simulink model "traffic_light"  (R2020a)
settings: Solver=VariableStepAuto  StartTime=0.0  StopTime=150  RelTol=1e-3
undefined symbols (not defined in the file): DiscIntNeverNeededParam
libraries: simulink x1
settings Model: Creator=Shubham  LastModifiedBy=Shubham

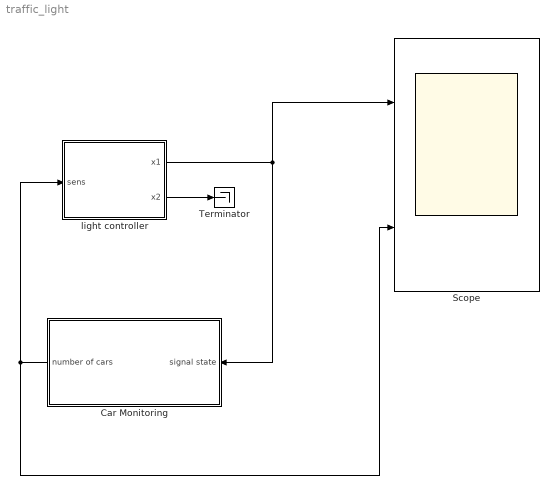
== system traffic_light ==
  Car Monitoring : Subsystem
  Scope : Scope  NumInputPorts=2
  Terminator : Terminator
  light controller : Stateflow chart  TreatAsAtomicUnit=on
  wires:
  light controller/2(x2) -> Terminator/1
  light controller/1(x1) -> Car Monitoring/1(signal state), Scope/1
  Car Monitoring/1(number of cars) -> light controller/1(sens), Scope/2

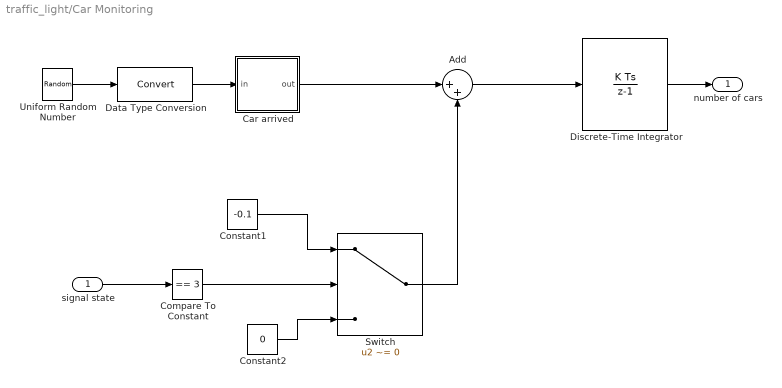
== system traffic_light/Car Monitoring ==
  signal state : Inport
  Add : Sum  Inputs=|++
  Car arrived : Stateflow chart  TreatAsAtomicUnit=on
  Compare To Constant : simulink/Logic and Bit Operations/Compare To Constant  relop===  const=3  OutDataTypeStr=boolean  ZeroCross=off
  Constant1 : Constant  Value=-0.1
  Constant2 : Constant  Value=0
  Data Type Conversion : DataTypeConversion
  Discrete-Time Integrator : DiscreteIntegrator  SampleTime=-1  LimitOutput=on  LowerSaturationLimit=0  ICPrevOutput=DiscIntNeverNeededParam  ICPrevScaledInput=DiscIntNeverNeededParam
  Switch : Switch  Criteria=u2 ~= 0
  Uniform Random Number : UniformRandomNumber  Minimum=0  Maximum=100  Seed=177836  SampleTime=0
  number of cars : Outport  VectorParamsAs1DForOutWhenUnconnected=off
  wires:
  Constant1/1 -> Switch/1
  Constant2/1 -> Switch/3
  Discrete-Time Integrator/1 -> number of cars/1
  signal state/1 -> Compare To Constant/1
  Compare To Constant/1 -> Switch/2
  Switch/1 -> Add/2
  Add/1 -> Discrete-Time Integrator/1
  Car arrived/1(out) -> Add/1
  Data Type Conversion/1 -> Car arrived/1(in)
  Uniform Random Number/1 -> Data Type Conversion/1

== stateflow chart traffic_light/light controller ==
  settings: stateMachineType=MOORE_MACHINE  executeAtInitialization=1  initializeOutput=1
  state Stop
    x1 = RED;
    x2 = GREEN;
  state StopForTraffic
    x1 = RED;
    x2 = GREEN;
  state StopToGo
    x1 = RED;
    x2 = YELLOW;
  state GoToStop
    x1 = YELLOW;
    x2 = RED;
  state Go
    x1 = GREEN;
    x2 = RED;
  (default) -> Stop
  StopForTraffic -> StopToGo : [sens]
  Stop -> StopForTraffic : after(25,tick)
  GoToStop -> Stop : after (7,tick)
  StopToGo -> Go : after(7,tick)
  Go -> GoToStop : after(10,tick)
  data: sens input double; RED constant uint8 =1; YELLOW constant double =2; GREEN constant double =3; x1 output double; x2 output double

== stateflow chart traffic_light/Car Monitoring/Car arrived ==
  (default) -> (junction 2) : {out = in > 90;}
  data: in input int8; out output double
